simulink model "Observable"  (Simulink 8.8)
settings: Solver=VariableStepAuto  StartTime=0.0  StopTime=10.0  RelTol=1e-3
settings Model: Creator=Bonner  LastModifiedBy=Administrator
settings DataIOCC: LimitDataPoints=off  SaveFormat=Dataset  SignalLoggingSaveFormat=Dataset
settings OptimizationCC: LifeSpan=auto
settings DebuggingCC: UnderspecifiedInitializationDetection=Simplified  MergeDetectMultiDrivingBlocksExec=error  FcnCallInpInsideContextMsg=error  StateNameClashWarn=none  SFUnexpectedBacktrackingDiag=error  SFNoUnconditionalDefaultTransitionDiag=error  SFExecutionAtInitializationDiag=warning
settings HardwareCC: ProdBitPerPointer=64  ProdBitPerSizeT=64  ProdBitPerPtrDiffT=64  ProdLargestAtomicFloat=Float  ProdIntDivRoundTo=Zero  ProdEndianess=LittleEndian  ProdWordSize=64  ProdHWDeviceType=Intel->x86-64 (Windows64)
settings ModelReferenceCC: PropagateSignalLabelsOutOfModel=on
settings GRTTargetCC: TargetLangStandard=C99 (ISO)  GeneratePreprocessorConditionals=Use local settings  CombineOutputUpdateFcns=on  GRTInterface=off
settings ConfigComp: CovMetricSettings=dwe  CovHtmlReporting=off  CovSaveCumulativeToWorkspaceVar=off  CovSaveSingleToWorkspaceVar=off  CovExternalEMLEnable=on

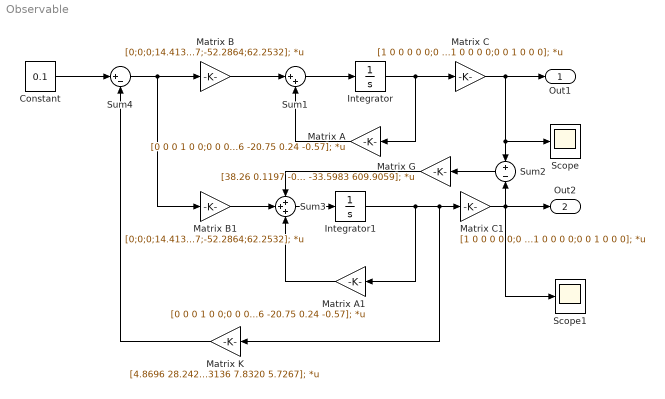
== system Observable ==
  Constant : Constant  Value=0.1
  Integrator : Integrator  InitialCondition=[0 0 0.1 0 0 0];
  Integrator1 : Integrator  InitialCondition=[0 0 0.1 0 0 0];  AbsoluteTolerance=0.001
  Matrix A : Gain  Gain=[0 0 0 1 0 0;0 0 0 0 1 0;0 0 0 0 0 1;0 -1.96 0.094 -4.8 0.004 -0.004;0 46.12 -25.01 18.76 -0.13 0.24;0 -51.01 78.16 -20.75 0.24 -0.57];  Multiplication=Matrix(K*u)
  Matrix A1 : Gain  Gain=[0 0 0 1 0 0;0 0 0 0 1 0;0 0 0 0 0 1;0 -1.96 0.094 -4.8 0.004 -0.004;0 46.12 -25.01 18.76 -0.13 0.24;0 -51.01 78.16 -20.75 0.24 -0.57];  Multiplication=Matrix(K*u)
  Matrix B : Gain  Gain=[0;0;0;14.4137;-52.2864;62.2532];  Multiplication=Matrix(K*u)
  Matrix B1 : Gain  Gain=[0;0;0;14.4137;-52.2864;62.2532];  Multiplication=Matrix(K*u)
  Matrix C : Gain  Gain=[1 0 0 0 0 0;0 1 0 0 0 0;0 0 1 0 0 0];  Multiplication=Matrix(K*u)
  Matrix C1 : Gain  Gain=[1 0 0 0 0 0;0 1 0 0 0 0;0 0 1 0 0 0];  Multiplication=Matrix(K*u)
  Matrix G : Gain  Gain=[38.26 0.1197 -0.2836;17.7903 44.7264 0.7555;-17.4652 0.6889 46.5137;275.9610 1.1437 -5.5261;690.8092 544.3198 -7.4808;-704.7150 -33.5983 609.9059];  Multiplication=Matrix(K*u)
  Matrix K : Gain  Gain=[4.8696 28.2425 36.0516 6.3136 7.8320 5.7267];  Multiplication=Matrix(K*u)
  Scope : Scope
  Scope1 : Scope
  Sum1 : Sum  Inputs=|++
  Sum2 : Sum  Inputs=+-
  Sum3 : Sum  Inputs=+++
  Sum4 : Sum  Inputs=|+-
  Out1 : Outport
  Out2 : Outport  Port=2
  wires:
  Constant/1 -> Sum4/1
  Matrix B/1 -> Sum1/1
  Sum1/1 -> Integrator/1
  Integrator/1 -> Matrix A/1, Matrix C/1
  Matrix C/1 -> Sum2/1, Scope/1, Out1/1
  Matrix A/1 -> Sum1/2
  Matrix B1/1 -> Sum3/2
  Matrix G/1 -> Sum3/1
  Sum3/1 -> Integrator1/1
  Sum2/1 -> Matrix G/1
  Integrator1/1 -> Matrix A1/1, Matrix K/1, Matrix C1/1
  Matrix C1/1 -> Scope1/1, Out2/1, Sum2/2
  Matrix A1/1 -> Sum3/3
  Matrix K/1 -> Sum4/2
  Sum4/1 -> Matrix B/1, Matrix B1/1
